simulink model "matprob2"  (R2020a)
settings: Solver=VariableStepAuto  StartTime=0.0  StopTime=10.0  RelTol=1e-3
settings Model: Creator=deepa  LastModifiedBy=deepa

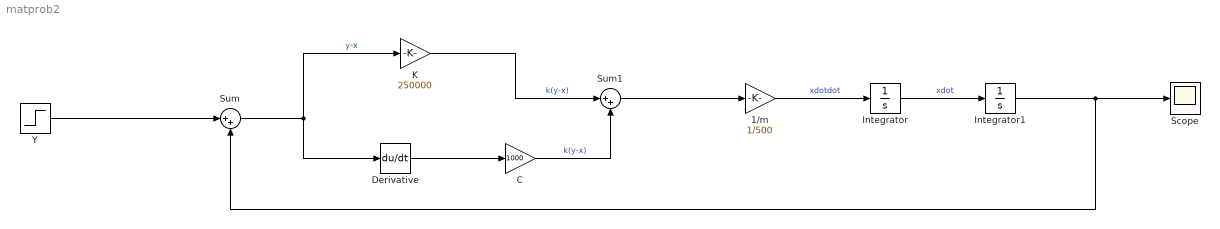
== system matprob2 ==
  1/m : Gain  Gain=1/500
  C : Gain  Gain=1000
  Derivative : Derivative
  Integrator : Integrator
  Integrator1 : Integrator
  K : Gain  Gain=250000
  Scope : Scope
  Sum : Sum  Inputs=|++
  Sum1 : Sum  Inputs=|++
  Y : Step  SampleTime=0
  wires:
  Y/1 -> Sum/1
  Sum/1 -> Derivative/1, K/1  "y-x"
  K/1 -> Sum1/1  "k(y-x)"
  Derivative/1 -> C/1
  C/1 -> Sum1/2  "k(y-x)"
  Sum1/1 -> 1/m/1
  1/m/1 -> Integrator/1  "xdotdot"
  Integrator/1 -> Integrator1/1  "xdot"
  Integrator1/1 -> Sum/2, Scope/1
